simulink model "MagnetoShield_PID_Nonlinear_Simulation_DT"  (R2019a)
settings: Solver=VariableStepAuto  StartTime=0.0  StopTime=15  RelTol=1e-3
undefined symbols (not defined in the file): C, g, Ke, Km, L, m, R, sigbuilder_block, Ts
libraries: simulink x1
settings Model: Creator=jakub  LastModifiedBy=jakub

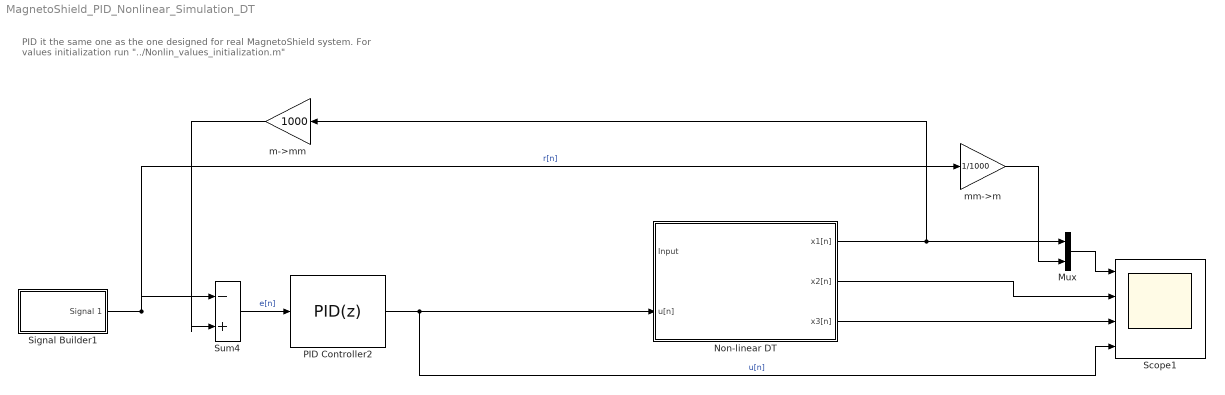
== system MagnetoShield_PID_Nonlinear_Simulation_DT ==
  note: PID it the same one as the one designed for real MagnetoShield system.
      | For values initialization run "../Nonlin_values_initialization.m"
  Mux : Mux  Inputs=2
  Non-linear DT : Subsystem
  PID Controller2 : simulink/Continuous/PID Controller  Controller=PID  Form=Ideal  TimeDomain=Discrete-time  SampleTime=Ts  IntegratorMethod=Forward Euler  FilterMethod=Forward Euler  ControllerParametersSource=internal  P=3.5  I=1/0.6  D=0.025  UseFilter=off  N=100  TunerSelectOption=Transfer Function Based (PID Tuner App)  InitialConditionSource=internal  InitialConditionForIntegrator=0  InitialConditionForFilter=0  DifferentiatorICPrevScaledInput=0  ExternalReset=none  TrackingMode=off  Kt=1  LimitOutput=on  UpperSaturationLimit=10  LowerSaturationLimit=0  LinearizeAsGain=on  AntiWindupMode=back-calculation  Kb=0.1  POutMin=[]  POutMax=[]  IOutMin=[]  IOutMax=[]  DOutMin=[]  DOutMax=[]  NOutMin=[]  NOutMax=[]  SumOutMin=[]  SumOutMax=[]  SaturationOutMin=[]  SaturationOutMax=[]  PParamMin=[]  PParamMax=[]  IParamMin=[]  IParamMax=[]  DParamMin=[]  DParamMax=[]  NParamMin=[]  NParamMax=[]  KbParamMin=[]  KbParamMax=[]  KtParamMin=[]  KtParamMax=[]  KbOutMin=[]  KbOutMax=[]  KtOutMin=[]  KtOutMax=[]  IntegratorOutMin=[]  IntegratorOutMax=[]  FilterOutMin=[]  FilterOutMax=[]  SumI1OutMin=[]  SumI1OutMax=[]  SumI2OutMin=[]  SumI2OutMax=[]  SumI3OutMin=[]  SumI3OutMax=[]  SumI4OutMin=[]  SumI4OutMax=[]  SumDOutMin=[]  SumDOutMax=[]  DifferentiatorOutMin=[]  DifferentiatorOutMax=[]  FilterDiffOutCoefMin=[]  FilterDiffOutCoefMax=[]  ReciprocalOutMin=[]  ReciprocalOutMax=[]  SumDenOutMin=[]  SumDenOutMax=[]  SumNumOutMin=[]  SumNumOutMax=[]  DivideOutMin=[]  DivideOutMax=[]  IntegratorContinuousStateAttributes=''  IntegratorStateMustResolveToSignalObject=off  IntegratorRTWStateStorageClass=Auto  FilterContinuousStateAttributes=''  FilterStateMustResolveToSignalObject=off  FilterRTWStateStorageClass=Auto  ParallelPVariant=Passthrough  IdealPVariant=InternalParameters  IVariant=InternalParameters  DVariant=InternalParameters  IntegratorVariant=Discrete  SatVariant=Enabled  AWVariant=BackCalculation  PCopyVariant=Disabled  TRVariant=Disabled  FdbkBlocksVariant=Forward  IdealPFdbkVariant=Disabled  SatFdbkVariant=Disabled  DerivativeFilterVariant=Differentiator  NVariant=Passthrough  NCopyVariant=Disabled_SignalSpec  FilterICVariant=InternalICsDifferentiator  IntegratorICVariant=InternalICs  ExternalResetVariant=Disabled  TRSumVariant=Passthrough  SumFdbkVariant=Disabled  SumVariant=Sum_PID
  Scope1 : Scope  NumInputPorts=4
  Signal Builder1 : Subsystem  Tag=STV Subsys  LoadFcn=sigbuilder_block('load');  StartFcn=sigbuilder_block('start');  StopFcn=sigbuilder_block('stop');  ClipboardFcn=sigbuilder_block('clipboard');  mask(Sigbuilder block){tuvar=[0:10]}
      mask help: Simulink:masks:SigbuilderBlock_MD
      mask init:
      | if ~strcmp(get_param(bdroot(gcbh),'SimulationStatus'),'stopped') tuvar = sigbuilder_block('maskInit'); end
      settings: CopyFcn=sigbuilder_block('copy');  DeleteFcn=sigbuilder_block('delete');  ModelCloseFcn=sigbuilder_block('modelClose');  PreSaveFcn=sigbuilder_block('preSave');  PauseFcn=sigbuilder_block('pause');  ContinueFcn=sigbuilder_block('continue');  NameChangeFcn=sigbuilder_block('namechange');  OpenFcn=sigbuilder_block('open',[434.4 169.8 550.8 400.2 ]);  CloseFcn=sigbuilder_block('close');
      mask Display: plot(0, 0, 100, 100,[2, 2, 32, 32, 2], [68, 8, 8, 68, 68],[32, 2], [38, 38], [32, 19, 2],[53, 60, 44], [32, 17, 17, 2],[16, 16, 31, 31]);txt = getActiveGroup(gcbh);text(2, 100, txt,'verticalAlignment', 'top');
  Sum4 : Sum  Inputs=|-+
  m->mm : Gain  Gain=1000
  mm->m : Gain  Gain=1/1000
  wires:
  Sum4/1 -> PID Controller2/1  "e[n]"
  PID Controller2/1 -> Non-linear DT/2(u[n]), Scope1/4  "u[n]"
  Non-linear DT/3(x3[n]) -> Scope1/3
  Signal Builder1/1(Signal 1) -> Sum4/1, mm->m/1  "r[n]"
  m->mm/1 -> Sum4/2
  Mux/1 -> Scope1/1
  mm->m/1 -> Mux/2
  Non-linear DT/2(x2[n]) -> Scope1/2
  Non-linear DT/1(x1[n]) -> Mux/1, m->mm/1

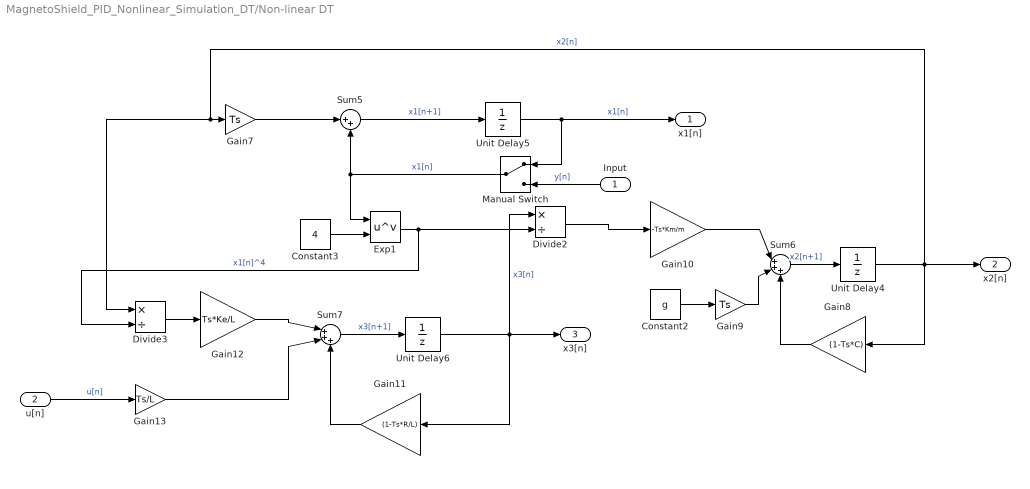
== system MagnetoShield_PID_Nonlinear_Simulation_DT/Non-linear DT ==
  Input : Inport
  u[n] : Inport  Port=2
  Constant2 : Constant  Value=g
  Constant3 : Constant  Value=4
  Divide2 : Product  Inputs=*/
  Divide3 : Product  Inputs=*/
  Exp1 : Math  Operator=pow  SaturateOnIntegerOverflow=on
  Gain10 : Gain  Gain=-Ts*Km/m
  Gain11 : Gain  Gain=(1-Ts*R/L)
  Gain12 : Gain  Gain=Ts*Ke/L
  Gain13 : Gain  Gain=Ts/L
  Gain7 : Gain  Gain=Ts
  Gain8 : Gain  Gain=(1-Ts*C)
  Gain9 : Gain  Gain=Ts
  Manual Switch : ManualSwitch
  Sum5 : Sum  Inputs=|++
  Sum6 : Sum  Inputs=|+++
  Sum7 : Sum  Inputs=|+++
  Unit Delay4 : UnitDelay  SampleTime=-1  HasFrameUpgradeWarning=on
  Unit Delay5 : UnitDelay  InitialCondition=0.017  SampleTime=-1  HasFrameUpgradeWarning=on
  Unit Delay6 : UnitDelay  SampleTime=-1  HasFrameUpgradeWarning=on
  x1[n] : Outport
  x2[n] : Outport  Port=2
  x3[n] : Outport  Port=3
  wires:
  Gain11/1 -> Sum7/3
  Gain13/1 -> Sum7/2
  Unit Delay6/1 -> Gain11/1, x3[n]/1, Divide2/1  "x3[n]"
  Gain9/1 -> Sum6/2
  Exp1/1 -> Divide3/2, Divide2/2  "x1[n]^4"
  Sum6/1 -> Unit Delay4/1  "x2[n+1]"
  Divide3/1 -> Gain12/1
  Gain12/1 -> Sum7/1
  Constant3/1 -> Exp1/2
  Constant2/1 -> Gain9/1
  u[n]/1 -> Gain13/1  "u[n]"
  Gain10/1 -> Sum6/1
  Unit Delay4/1 -> Divide3/1, Gain7/1, x2[n]/1, Gain8/1  "x2[n]"
  Sum7/1 -> Unit Delay6/1  "x3[n+1]"
  Gain8/1 -> Sum6/3
  Gain7/1 -> Sum5/1
  Divide2/1 -> Gain10/1
  Sum5/1 -> Unit Delay5/1  "x1[n+1]"
  Unit Delay5/1 -> x1[n]/1, Manual Switch/1  "x1[n]"
  Manual Switch/1 -> Exp1/1, Sum5/2  "x1[n]"
  Input/1 -> Manual Switch/2  "y[n]"

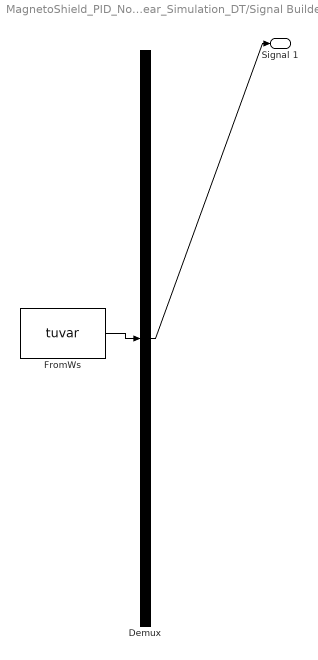
== system MagnetoShield_PID_Nonlinear_Simulation_DT/Signal Builder1 ==
  Demux : Demux  Tag=STV Demux  Outputs=1
  FromWs : FromWorkspace  Tag=STV FromWs  VariableName=tuvar  SampleTime=0
      SigBuilderData=|
      | common.afterFinalStr = 'Extrapolate'
      | common.sampleTime = 0
      | dataSet.timeRange = [0 15]
      | dataSet.name = 'Group 1'
      | sbobj.Groups.Name = 'Group 1'
      | sbobj.Groups.Signals.Name = 'Signal 1'
      | sbobj.Groups.Signals.XData = [0 2 2 4 4 6 6 8 10 12 14 14 15]
      | sbobj.Groups.Signals.YData = [15.5 15.5 14 14 12.5 12.5 14.5 14.5 17 12 14.5 16 16]
      | sbobj.Groups.TimeRange = [0 15]
  Signal 1 : Outport  Tag=STV Outport
  wires:
  FromWs/1 -> Demux/1
  Demux/1 -> Signal 1/1
